simulink model "simulation_matlab2"  (R2021b)
settings: Solver=VariableStepAuto  StartTime=0.0  StopTime=10  RelTol=1e-3
InitFcn:
  | Rm=3.15;
  | Lm=0.0015;
  | K=1.028;
  | fm=0.16805;
  | A2=0.0033153;
  | A1=0.045721;
  | L01=0.2625;
  | m2=0.24355;
  | A1tilde=A1+A2+m2*L01*L01;
  | A2tilde=A1tilde-A2;
  | f=0.070633;
  | lg1=0.16655703376925832;
  | m1=0.66984;
  | g=9.8;
  | Ceq=L01*m2*g+lg1*m1*g;
settings Model: PauseTimes=1  Creator=mimom  LastModifiedBy=dviol
settings DebuggingCC: UnconnectedInputMsg=none  UnconnectedOutputMsg=none  UnconnectedLineMsg=none
settings ModelReferenceCC: EnableRefExpFcnMdlSchedulingChecks=off
settings RTWCC: DLArmComputeVersion=20.02.1

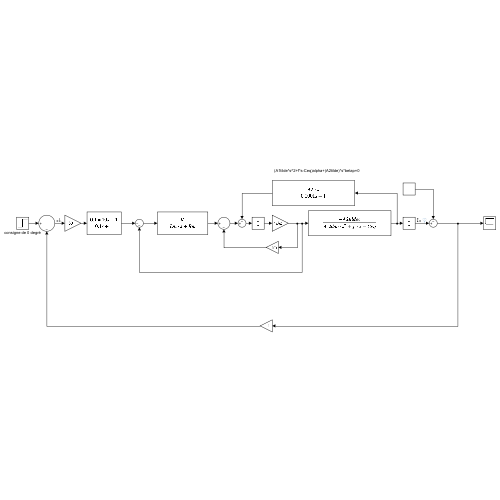
[thumbnail: Simulink's stored preview of the top-level diagram]
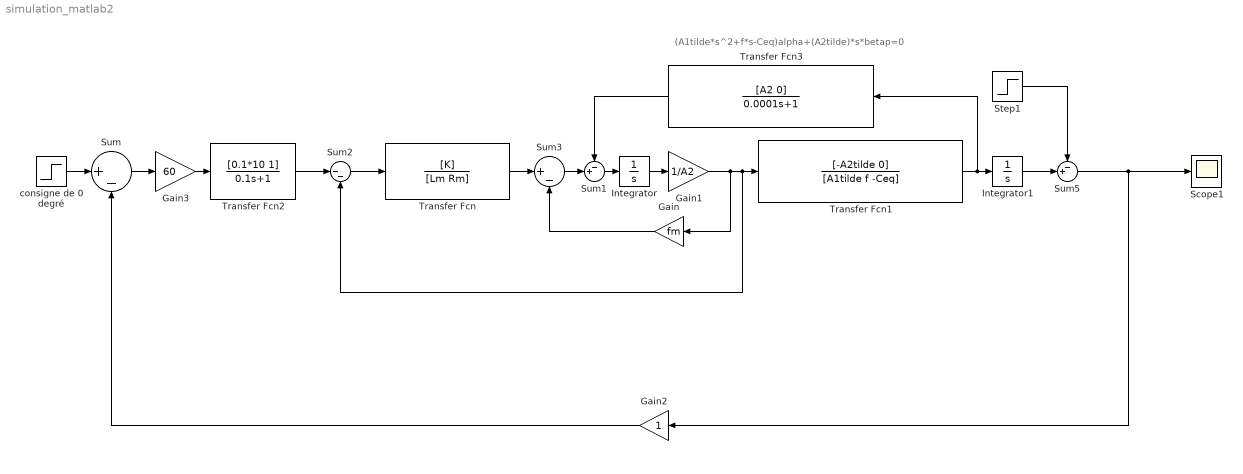
== system simulation_matlab2 ==
  note: (A1tilde*s^2+f*s-Ceq)alpha+(A2tilde)*s*betap=0
  Gain : Gain  Gain=fm
  Gain1 : Gain  Gain=1/A2
  Gain2 : Gain
  Gain3 : Gain  Gain=60
  Integrator : Integrator
  Integrator1 : Integrator
  Scope1 : Scope
  Step1 : Step  Time=0  After=-0.1  SampleTime=0
  Sum : Sum  Inputs=|+-
  Sum1 : Sum  Inputs=-+|
  Sum2 : Sum  Inputs=|--
  Sum3 : Sum  Inputs=|+-
  Sum5 : Sum  Inputs=-+|
  Transfer Fcn : TransferFcn  Numerator=[K]  Denominator=[Lm Rm]
  Transfer Fcn1 : TransferFcn  Numerator=[-A2tilde 0]  Denominator=[A1tilde f -Ceq]
  Transfer Fcn2 : TransferFcn  Numerator=[0.1*10 1]  Denominator=[0.1 1]
  Transfer Fcn3 : TransferFcn  Numerator=[A2 0]  Denominator=[0.0001 1]
  consigne de 0 degré : Step  Time=0  After=0.1  SampleTime=0
  wires:
  consigne de 0 degré/1 -> Sum/1
  Gain2/1 -> Sum/2
  Sum/1 -> Gain3/1
  Sum2/1 -> Transfer Fcn/1
  Transfer Fcn/1 -> Sum3/1
  Gain/1 -> Sum3/2
  Integrator/1 -> Gain1/1
  Step1/1 -> Sum5/1
  Sum5/1 -> Gain2/1, Scope1/1
  Integrator1/1 -> Sum5/2
  Transfer Fcn1/1 -> Transfer Fcn3/1, Integrator1/1
  Transfer Fcn2/1 -> Sum2/1
  Gain3/1 -> Transfer Fcn2/1
  Gain1/1 -> Sum2/2, Transfer Fcn1/1, Gain/1
  Sum3/1 -> Sum1/2
  Sum1/1 -> Integrator/1
  Transfer Fcn3/1 -> Sum1/1
